simulink model "Chopper_full_load_half_speed"  (R2024b)
settings: Solver=VariableStepAuto  StartTime=0.0  StopTime=30  RelTol=1e-3
values from neighbouring files (symbols this model uses):
  imax = Tl/ke    (= 780.373749459)    [Chopper_full_load_half_speed1.m]
  J = 5    [Chopper_full_load_half_speed1.m]
  ke = 3.65    [Chopper_full_load_half_speed1.m]
  Kii = wbwi*Ra/Vg    (= 0.163362817987)    [Chopper_full_load_half_speed1.m]
  Kiw = J/(ke*Tfil*Tfil*a*a*a)    [Chopper_full_load_half_speed1.m]
  Kpi = Kii*La/Ra    (= 0.00314159265359)    [Chopper_full_load_half_speed1.m]
  Kpw = J/(ke*Tfil*a)    [Chopper_full_load_half_speed1.m]
  La = 0.001    [Chopper_full_load_half_speed1.m]
  Ra = 0.052    [Chopper_full_load_half_speed1.m]
  T = Tl    (= 2848.36418553)    [Chopper_full_load_half_speed1.m]
  Tfil = 1/20    (= 0.05)    [Chopper_full_load_half_speed1.m]
  Vg = 800    [Chopper_full_load_half_speed1.m]
  W = 625    [Chopper_full_load_half_speed1.m]
libraries: spsIGBTDiodeLib x4, spsDCMachineLib x1, spsDCVoltageSourceLib x1, spsTriangleGeneratorLib x1, sps_lib x1
settings Model: LastModifiedBy=PREKSHA

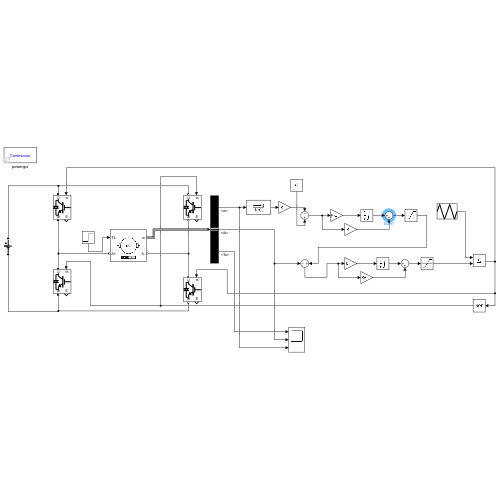
[thumbnail: Simulink's stored preview of the top-level diagram]
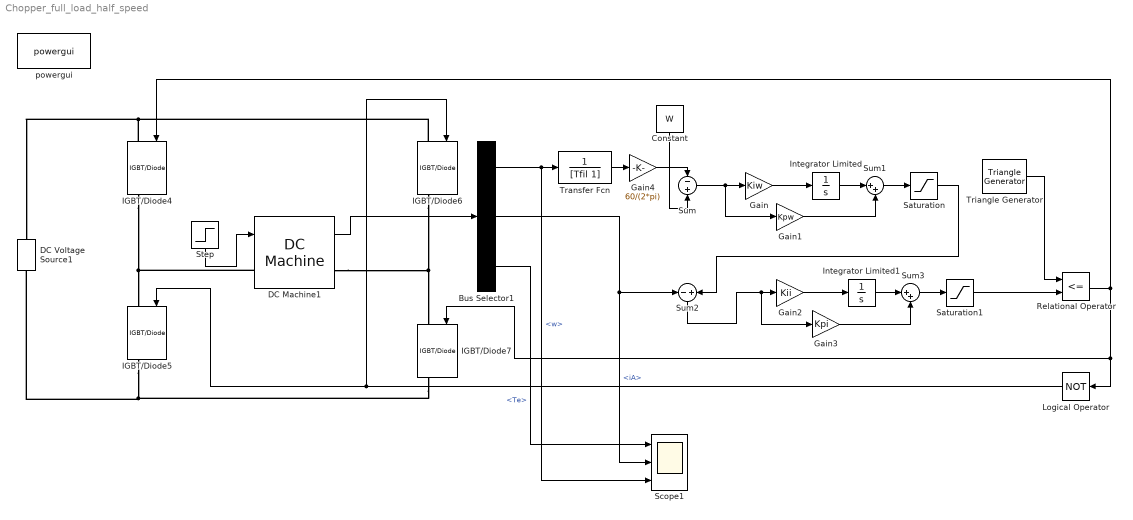
== system Chopper_full_load_half_speed ==
  Bus Selector1 : BusSelector  OutputSignals=w,iA,Te
  Constant : Constant  Value=W
  DC Machine1 : spsDCMachineLib/DC Machine  PresetModel=No  MechanicalLoad=Torque TL  FieldType=Permanent magnet  ShowDetailedParameters=on  MeasurementBus=on  RLa="[ Ra  La]"  RLf="[ 240  120]"  Laf=1.8  MachineConstant=Torque constant (N.m/A)  Ke=1.8  Kt=ke  J=J  Bm=0  Tf=0  w0=1  Ifinit=1  TsPowergui=0  TsBlock=-1
  DC Voltage Source1 : spsDCVoltageSourceLib/DC Voltage Source  Amplitude=Vg  Measurements=None
  Gain : Gain  Gain=Kiw
  Gain1 : Gain  Gain=Kpw
  Gain2 : Gain  Gain=Kii
  Gain3 : Gain  Gain=Kpi
  Gain4 : Gain  Gain=60/(2*pi)
  IGBT/Diode{4..7} (4 alike) : spsIGBTDiodeLib/IGBT//Diode  Ron=1e-3  Rs=1e5  Cs=inf  Measurements=on
  Integrator Limited : Integrator  LimitOutput=on  UpperSaturationLimit=imax  LowerSaturationLimit=-imax
  Integrator Limited1 : Integrator  LimitOutput=on  UpperSaturationLimit=1  LowerSaturationLimit=-1
  Logical Operator : Logic  Operator=NOT  AllPortsSameDT=off  OutDataTypeStr=boolean
  Relational Operator : RelationalOperator  Operator=<=  OutDataTypeStr=boolean  RndMeth=Simplest  InputSameDT=off
  Saturation : Saturate  UpperLimit=imax  LowerLimit=-imax
  Saturation1 : Saturate  UpperLimit=1  LowerLimit=-1
  Scope1 : Scope  NumInputPorts=3
  Step : Step  Time=0.25  After=T  SampleTime=0
  Sum : Sum  Inputs=-+
  Sum1 : Sum  Inputs=|++
  Sum2 : Sum  Inputs=-+
  Sum3 : Sum  Inputs=|++
  Transfer Fcn : TransferFcn  Denominator=[Tfil 1]
  Triangle Generator : spsTriangleGeneratorLib/Triangle Generator  Freq=fsw  Phase=90  Ts=0
  powergui : sps_lib/powergui  Priority=1  SimulationMode=Continuous  SampleTime=50e-6  frequency=60  Iterations=50  frequencyindice=0  Pbase=100e6  ErrMax=1e-4  UnitsV=kV  UnitsW=MW  buscounter=0  FunctionMessages=off  echomessages=off  EnableUseOfTLC=off  CurrentSourceSwitches=off  DisableSnubberDevices=off  DisableRonSwitches=off  DisableVfSwitches=off  DisplayEquations=off  AutomaticDiscreteSolvers=off  SolverType=Tustin/Backward Euler (TBE)  Interpol=off  ExternalGateDelay=off  methode=off  Ts=100  x0status=blocks  SPID=on  SwTol=0  HookPort=off  NonlinearTolerance=1e-4  nMaxIteration=100  ContinueOnMaxIteration=off  RestoreLinks=warning  ResistiveCurrentMeasurement=off  Frange=[0:2:500]  Ylog=off  Xlog=on  ShowGrid=off  save=off  variable=ZData  structure=0  ZoomFFT=off  StartTime=0.0  cycles=1  DisplayStyle=1  fundamental=60  FreqAxis=off  MaxFrequency=1000  frequencyindicesteady=1  RmsSteady=1  display=off
  wires:
  DC Machine1/1 -> Bus Selector1/1
  Constant/1 -> Sum/2
  Sum/1 -> Gain1/1, Gain/1
  Gain/1 -> Integrator Limited/1
  Integrator Limited/1 -> Sum1/1
  Gain1/1 -> Sum1/2
  Sum1/1 -> Saturation/1
  Bus Selector1/2 -> Scope1/2, Sum2/1  "<iA>"
  Sum2/1 -> Gain3/1, Gain2/1
  Gain3/1 -> Sum3/2
  Gain2/1 -> Integrator Limited1/1
  Sum3/1 -> Saturation1/1
  Integrator Limited1/1 -> Sum3/1
  Saturation/1 -> Sum2/2
  Saturation1/1 -> Relational Operator/2
  Triangle Generator/1 -> Relational Operator/1
  Relational Operator/1 -> IGBT/Diode4/1, IGBT/Diode7/1, Logical Operator/1
  Logical Operator/1 -> IGBT/Diode5/1, IGBT/Diode6/1
  Gain4/1 -> Sum/1
  Bus Selector1/3 -> Scope1/1  "<Te>"
  Bus Selector1/1 -> Transfer Fcn/1, Scope1/3  "<w>"
  Transfer Fcn/1 -> Gain4/1
  Step/1 -> DC Machine1/1
  connections:
  IGBT/Diode4/RConn1 -- DC Machine1/LConn1 -- IGBT/Diode5/LConn1
  IGBT/Diode4/LConn1 -- IGBT/Diode6/LConn1 -- DC Voltage Source1/RConn1
  IGBT/Diode5/RConn1 -- IGBT/Diode7/RConn1 -- DC Voltage Source1/LConn1
  IGBT/Diode6/RConn1 -- DC Machine1/RConn1 -- IGBT/Diode7/LConn1
